simulink model "case_9_both_stopped_gap_too_big"  (R2025a)
settings: Solver=VariableStepAuto  StartTime=0.0  StopTime=10.0  RelTol=1e-3
settings Model: Creator=sanborkl  LastModifiedBy=sanborkl

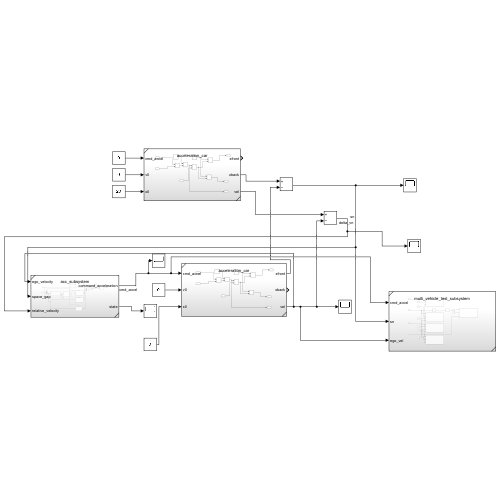
[thumbnail: Simulink's stored preview of the top-level diagram]
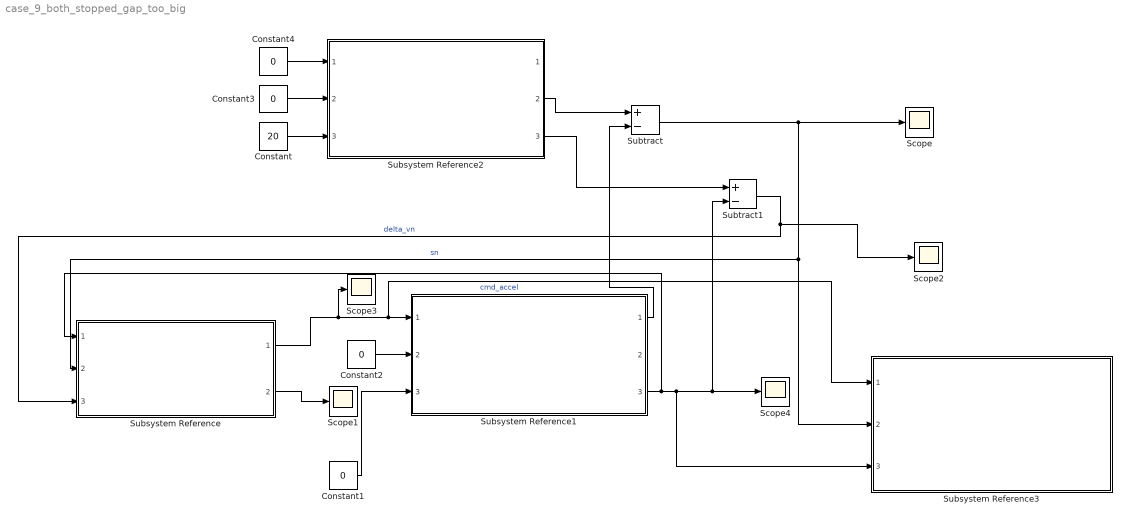
== system case_9_both_stopped_gap_too_big ==
  Constant : Constant  Value=20
  Constant{1..4} (4 alike) : Constant  Value=0
  Scope{,1..4} (5 alike) : Scope
      Scope settings: ActiveDisplayYMinimum=-1.8340687344850353  ActiveDisplayYMaximum=17.714896526053892
      Scope1 settings: ActiveDisplayYMinimum=-0.24999999999999994  ActiveDisplayYMaximum=2.25  DataLoggingVariableName=ScopeData2
      Scope2 settings: ActiveDisplayYMinimum=-5.2891527550196917  ActiveDisplayYMaximum=1.0122991772832779  DataLoggingVariableName=ScopeData3
      Scope3 settings: ActiveDisplayYMinimum=-2.6168604470924368  ActiveDisplayYMaximum=2.1364871313349303  DataLoggingVariableName=ScopeData4
      Scope4 settings: ActiveDisplayYMinimum=-0.571560265968523  ActiveDisplayYMaximum=5.1440423937167088
  Subsystem Reference : Subsystem  ReferencedSubsystem=acc_subsystem
  Subsystem Reference1 : Subsystem  ReferencedSubsystem=acceleration_car
  Subsystem Reference2 : Subsystem  ReferencedSubsystem=acceleration_car
  Subsystem Reference3 : Subsystem  ReferencedSubsystem=multi_vehicle_test_subsystem
  Subtract : Sum  Inputs=+-
  Subtract1 : Sum  Inputs=+-
  wires:
  Constant4/1 -> Subsystem Reference2/1
  Subsystem Reference2/3 -> Subtract1/1
  Subsystem Reference/1 -> Scope3/1, Subsystem Reference3/1, Subsystem Reference1/1  "cmd_accel"
  Constant3/1 -> Subsystem Reference2/2
  Constant2/1 -> Subsystem Reference1/2
  Subsystem Reference/2 -> Scope1/1
  Constant/1 -> Subsystem Reference2/3
  Subsystem Reference1/1 -> Subtract/2
  Subsystem Reference2/2 -> Subtract/1
  Subsystem Reference1/3 -> Subsystem Reference/1, Subsystem Reference3/3, Subtract1/2, Scope4/1
  Subtract1/1 -> Scope2/1, Subsystem Reference/3  "delta_vn"
  Subtract/1 -> Subsystem Reference3/2, Subsystem Reference/2, Scope/1  "sn"
  Constant1/1 -> Subsystem Reference1/3
